simulink model "TO20SpeedController"  (Simulink 8.2)
settings: Solver=ode45  StartTime=0.0  StopTime=150  RelTol=1e-3
libraries: simulink x2
settings Model: Creator=leslieem  LastModifiedBy=leslieem
settings DataIOCC: SignalLoggingSaveFormat=Dataset
settings OptimizationCC: ExpressionDepthLimit=128
settings DebuggingCC: FcnCallInpInsideContextMsg=EnableAllAsError  StateNameClashWarn=none
settings GRTTargetCC: CombineOutputUpdateFcns=on  GRTInterface=off

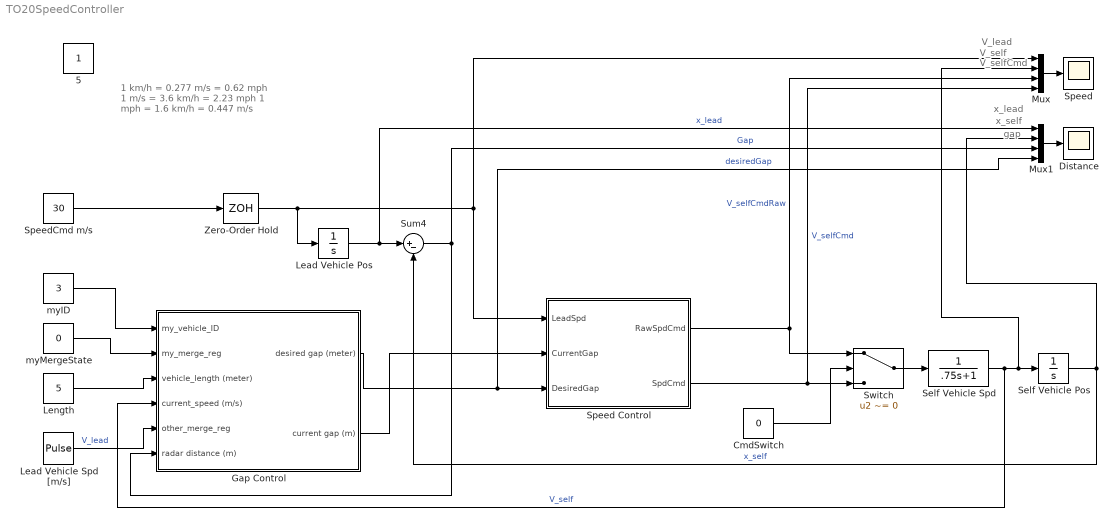
== system TO20SpeedController ==
  note: 1 km/h = 0.277 m/s = 0.62 mph
      | 1 m/s = 3.6 km/h = 2.23 mph
      | 1 mph = 1.6 km/h = 0.447 m/s
  note: V_lead
  note: V_selfCmd
  note: x_self
  note: x_lead
  note: V_self
  note: gap
  CmdSwitch : Constant  Value=0
  Distance : Scope
      settings: ShowLegends=on  YMax=200  MaxDataPoints=15000
  Gap Control : Subsystem
  Lead Vehicle Pos : Integrator  InitialCondition=10
  Lead Vehicle Spd [m/s] : DiscretePulseGenerator  PulseType=Time based  Period=180  PulseWidth=50  PhaseDelay=20
  Length : Constant  Value=5
  Mux : Mux
  Mux1 : Mux
  Self Vehicle Pos : Integrator
  Self Vehicle Spd : TransferFcn  Denominator=[.75 1]
  Speed : Scope
      settings: ShowLegends=on  YMax=35  MaxDataPoints=15000
  Speed Control : Subsystem
  SpeedCmd m/s : Constant  Value=30
  Sum4 : Sum  Inputs=|+-
  Switch : Switch  Criteria=u2 ~= 0
  Zero-Order Hold : ZeroOrderHold  SampleTime=0.01
  myID : Constant  Value=3
  myMergeState : Constant  Value=0
  5 : Constant  IOType=siggen
  wires:
  Mux/1 -> Speed/1
  Self Vehicle Pos/1 -> Mux1/2, Sum4/2  "x_self"
  Mux1/1 -> Distance/1
  Sum4/1 -> Gap Control/6(radar distance (m)), Mux1/3  "Gap"
  Self Vehicle Spd/1 -> Gap Control/4(current_speed (m/s)), Mux/2, Self Vehicle Pos/1  "V_self"
  Zero-Order Hold/1 -> Lead Vehicle Pos/1, Mux/1, Speed Control/1(LeadSpd)
  Speed Control/1(RawSpdCmd) -> Mux/3, Switch/1  "V_selfCmdRaw"
  Lead Vehicle Pos/1 -> Sum4/1, Mux1/1  "x_lead"
  Gap Control/1(desired gap (meter)) -> Speed Control/3(DesiredGap), Mux1/4  "desiredGap"
  SpeedCmd m/s/1 -> Zero-Order Hold/1
  Lead Vehicle Spd [m/s]/1 -> Gap Control/5(other_merge_reg)  "V_lead"
  Length/1 -> Gap Control/3(vehicle_length (meter))
  myMergeState/1 -> Gap Control/2(my_merge_reg)
  myID/1 -> Gap Control/1(my_vehicle_ID)
  Speed Control/2(SpdCmd) -> Mux/4, Switch/3  "V_selfCmd"
  Switch/1 -> Self Vehicle Spd/1
  CmdSwitch/1 -> Switch/2
  Gap Control/2(current gap (m)) -> Speed Control/2(CurrentGap)

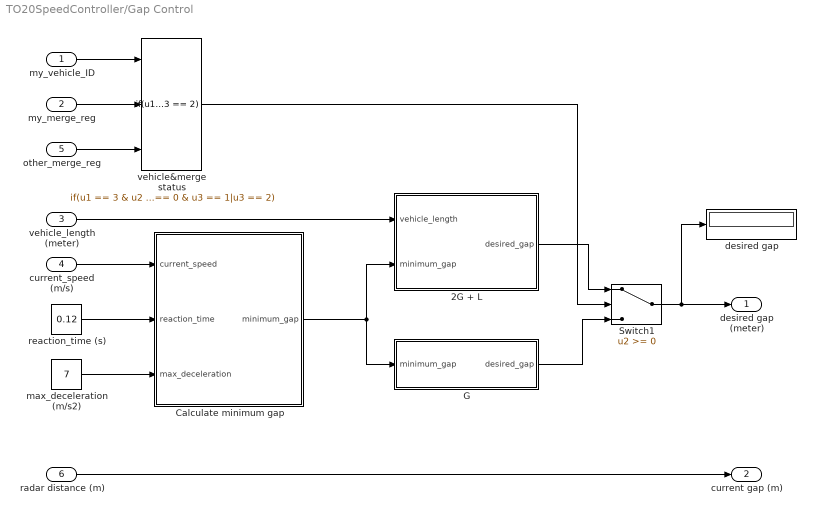
== system TO20SpeedController/Gap Control ==
  my_vehicle_ID : Inport
  my_merge_reg : Inport  Port=2
  vehicle_length (meter) : Inport  Port=3
  current_speed (m/s) : Inport  Port=4
  other_merge_reg : Inport  Port=5
  radar distance (m) : Inport  Port=6
  2G + L : Subsystem  TreatAsAtomicUnit=on
  Calculate minimum gap : Subsystem
  G : Subsystem  TreatAsAtomicUnit=on
  Switch1 : Switch
  desired gap : Display
  max_deceleration (m/s2) : Constant  Value=7
  reaction_time (s) : Constant  Value=0.12
  vehicle&merge status : If  NumInputs=3  IfExpression=u1 == 3 & u2 == 0 & u3 == 1|u3 == 2  ShowElse=off
  desired gap (meter) : Outport
  current gap (m) : Outport  Port=2
  wires:
  Switch1/1 -> desired gap/1, desired gap (meter)/1
  G/1(desired_gap) -> Switch1/3
  2G + L/1(desired_gap) -> Switch1/1
  Calculate minimum gap/1(minimum_gap) -> 2G + L/2(minimum_gap), G/1(minimum_gap)
  vehicle&merge status/1 -> Switch1/2
  max_deceleration (m/s2)/1 -> Calculate minimum gap/3(max_deceleration)
  reaction_time (s)/1 -> Calculate minimum gap/2(reaction_time)
  other_merge_reg/1 -> vehicle&merge status/3
  my_merge_reg/1 -> vehicle&merge status/2
  my_vehicle_ID/1 -> vehicle&merge status/1
  current_speed (m/s)/1 -> Calculate minimum gap/1(current_speed)
  vehicle_length (meter)/1 -> 2G + L/1(vehicle_length)
  radar distance (m)/1 -> current gap (m)/1

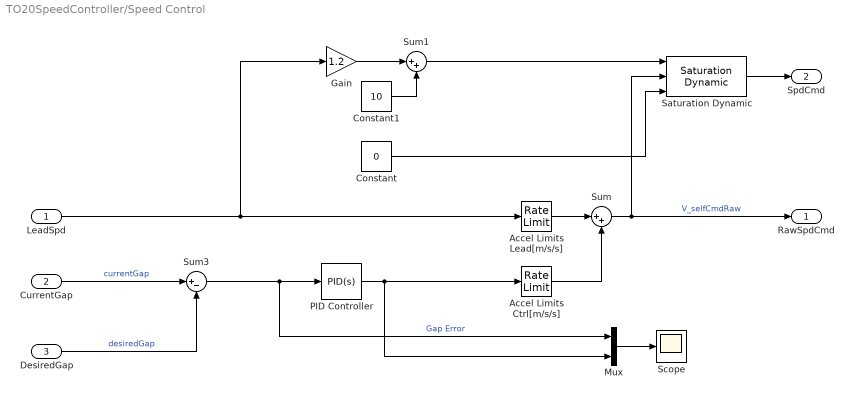
== system TO20SpeedController/Speed Control ==
  LeadSpd : Inport
  CurrentGap : Inport  Port=2
  DesiredGap : Inport  Port=3
  Accel Limits Ctrl[m/s/s] : RateLimiter  RisingSlewLimit=3  FallingSlewLimit=-3  SampleTimeMode=inherited
  Accel Limits Lead[m/s/s] : RateLimiter  RisingSlewLimit=5  FallingSlewLimit=-20  SampleTimeMode=inherited
  Constant : Constant  Value=0
  Constant1 : Constant  Value=10
  Gain : Gain  Gain=1.2
  Mux : Mux  Inputs=2
  PID Controller : simulink/Continuous/PID Controller  Controller=PID  TimeDomain=Continuous-time  SampleTime=1  IntegratorMethod=Forward Euler  FilterMethod=Forward Euler  Form=Parallel  P=1  I=0.1  D=0.01  N=100  InitialConditionSource=internal  InitialConditionForIntegrator=0  InitialConditionForFilter=0  ExternalReset=none  LimitOutput=on  UpperSaturationLimit=12  LowerSaturationLimit=-12  LinearizeAsGain=on  AntiWindupMode=back-calculation  Kb=1  TrackingMode=off  Kt=1  PParamMin=[]  PParamMax=[]  IParamMin=[]  IParamMax=[]  DParamMin=[]  DParamMax=[]  NParamMin=[]  NParamMax=[]  KbParamMin=[]  KbParamMax=[]  KtParamMin=[]  KtParamMax=[]  POutMin=[]  POutMax=[]  IOutMin=[]  IOutMax=[]  DOutMin=[]  DOutMax=[]  NOutMin=[]  NOutMax=[]  KbOutMin=[]  KbOutMax=[]  KtOutMin=[]  KtOutMax=[]  IntegratorOutMin=[]  IntegratorOutMax=[]  FilterOutMin=[]  FilterOutMax=[]  SumOutMin=[]  SumOutMax=[]  SumI1OutMin=[]  SumI1OutMax=[]  SumI2OutMin=[]  SumI2OutMax=[]  SumI3OutMin=[]  SumI3OutMax=[]  SumDOutMin=[]  SumDOutMax=[]  SaturationOutMin=[]  SaturationOutMax=[]  IntegratorContinuousStateAttributes=''  IntegratorStateMustResolveToSignalObject=off  IntegratorRTWStateStorageClass=Auto  FilterContinuousStateAttributes=''  FilterStateMustResolveToSignalObject=off  FilterRTWStateStorageClass=Auto
  Saturation Dynamic : simulink/Discontinuities/Saturation Dynamic  OutMin=[]  OutMax=[]  OutDataTypeStr=Inherit: Same as second input  OutDataType=fixdt(1, 16)  OutScaling=2^-10  DoSatur=off
  Scope : Scope
      settings: ShowLegends=on  YMin=-50  YMax=50  SaveName=ScopeData2  MaxDataPoints=15000
  Sum : Sum  Inputs=|++
  Sum1 : Sum  Inputs=|++
  Sum3 : Sum  Inputs=|+-
  RawSpdCmd : Outport
  SpdCmd : Outport  Port=2
  wires:
  Sum3/1 -> PID Controller/1, Mux/1  "Gap Error"
  DesiredGap/1 -> Sum3/2  "desiredGap"
  LeadSpd/1 -> Gain/1, Accel Limits Lead[m/s/s]/1
  Mux/1 -> Scope/1
  CurrentGap/1 -> Sum3/1  "currentGap"
  Sum/1 -> RawSpdCmd/1, Saturation Dynamic/2  "V_selfCmdRaw"
  Constant/1 -> Saturation Dynamic/3
  Sum1/1 -> Saturation Dynamic/1
  Gain/1 -> Sum1/1
  Constant1/1 -> Sum1/2
  Saturation Dynamic/1 -> SpdCmd/1
  Accel Limits Ctrl[m/s/s]/1 -> Sum/2
  Accel Limits Lead[m/s/s]/1 -> Sum/1
  PID Controller/1 -> Accel Limits Ctrl[m/s/s]/1, Mux/2

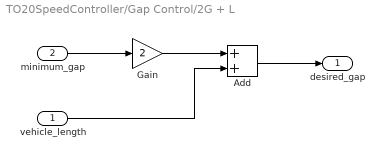
== system TO20SpeedController/Gap Control/2G + L ==
  vehicle_length : Inport
  minimum_gap : Inport  Port=2
  Add : Sum
  Gain : Gain  Gain=2
  desired_gap : Outport
  wires:
  Add/1 -> desired_gap/1
  vehicle_length/1 -> Add/2
  Gain/1 -> Add/1
  minimum_gap/1 -> Gain/1

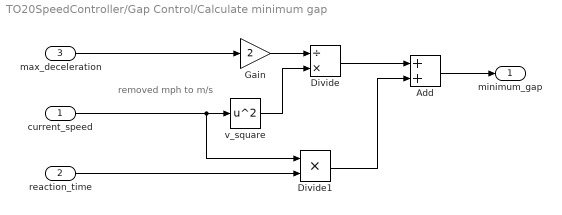
== system TO20SpeedController/Gap Control/Calculate minimum gap ==
  note: removed mph to m/s
  current_speed : Inport
  reaction_time : Inport  Port=2
  max_deceleration : Inport  Port=3
  Add : Sum
  Divide : Product  Inputs=/*
  Divide1 : Product  Inputs=**
  Gain : Gain  Gain=2
  v_square : Math  Operator=square  SaturateOnIntegerOverflow=on
  minimum_gap : Outport
  wires:
  current_speed/1 -> v_square/1, Divide1/1
  reaction_time/1 -> Divide1/2
  v_square/1 -> Divide/2
  max_deceleration/1 -> Gain/1
  Gain/1 -> Divide/1
  Add/1 -> minimum_gap/1
  Divide1/1 -> Add/2
  Divide/1 -> Add/1

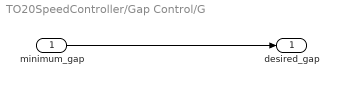
== system TO20SpeedController/Gap Control/G ==
  minimum_gap : Inport
  desired_gap : Outport
  wires:
  minimum_gap/1 -> desired_gap/1
